simulink model "AutoDriveTest"  (R2023a)
settings: Solver=FixedStepDiscrete  StartTime=0.0  StopTime=10.0  RelTol=1e-3
model workspace (MAT data in the model file):
  firstWarning = 1
  originalScenarioChecksum = '0FA6558D509BC7BD481F436FBA94739B'
libraries: sim3dlib x1, sim3dautolib x1
settings Model: Creator=Franz  LastModifiedBy=Franz

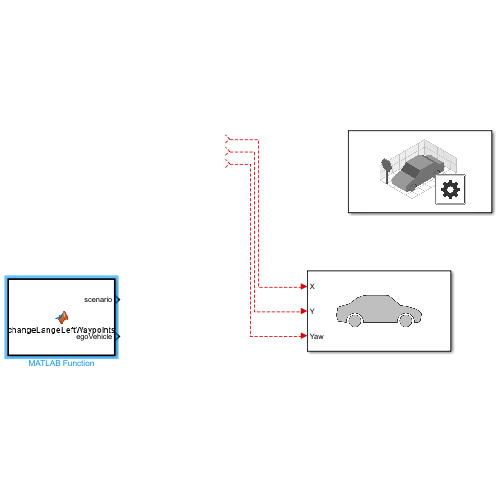
[thumbnail: Simulink's stored preview of the top-level diagram]
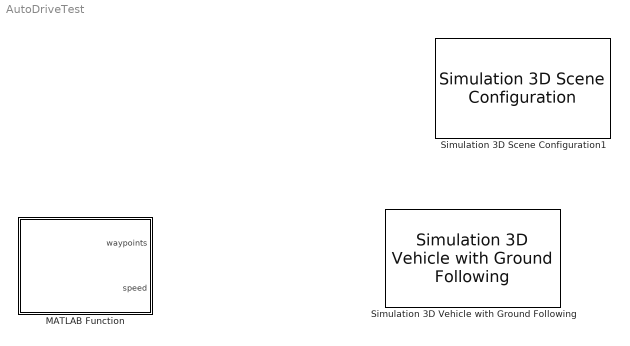
== system AutoDriveTest ==
  MATLAB Function : MATLAB Function  TreatAsAtomicUnit=on
  Simulation 3D Scene Configuration1 : sim3dlib/Simulation 3D Scene Configuration  Priority=0  ProjectFormat=Default Scenes  SceneDesc=Straight road  ProjectName=D:\Program Files\MATLAB\R2023a\toolbox\shared\sim3d_projects\automotive_project\UE4\WindowsNoEditor\VehicleSimulation.exe  ScenePath=/Game/Maps/HwStrght  EnableOpenDRIVE=off  vehTagList={'Scene Origin';'SimulinkVehicle1'}  vehTag=SimulinkVehicle1  OpVisEn=off  Ts=1/60  EnableWindow=off  EnableRemoteAccess=off  EnableWeather=off  SunAltitude=40.0  SunAzimuth=90  clouds=10  wind=1  fog=0  rain=0  EnableGeospatial=off  OriginHeight=200  OriginLatitude=40.744652  OriginLongitude=-73.988864  MapStyle=Aerial  AdditionalAssetIDs=[]  UseAdvancedSunSky=off  SolarTime=11  TimeZone=-5  Day=21  Month=9  Year=2022  UseDaylightSavingTime=on  DSTStartDay=10  DSTStartMonth=3  DSTEndDay=3  DSTEndMonth=11  DSTSwitchHour=2  sensorTag=MainCamera1  sensorId=1  sensorName=MainCamera1  mountLoc=Origin  offsetFlag=off  tmountOffset=[0, 0, 0]  rmountOffset=[0, 0, 0]  HorizontalResolution=1280  VerticalResolution=720  HorizontalFOV=60  mountPoint=[0 0 0]  mountOrientation=[0 0 0]  aMode=3  ID=1  GeoTrigger=Inactive
      settings: LibrarySourceBlock=drivingsim3d/Simulation 3D Scene Configuration
  Simulation 3D Vehicle with Ground Following : sim3dautolib/Simulation 3D Vehicle with Ground Following  Priority=-1  PassVehMesh=Muscle car  MeshPath=/MathWorksAutomotiveContent/Vehicles/Muscle/Meshes/SK_MuscleCar.SK_MuscleCar  TrackWidth=1.9  WheelBase=3  WheelRadius=0.35  VehColor=Red  InitialPos=[0, 0, 0]  InitialRot=[0, 0, 0]  ActorName=SimulinkVehicle1  SampleTime=-1  ActorType=SimulinkVehicle  ID=1  aMode=3  ActorTag=SimulinkVehicle1  CoordinateScheme=ISO  VehLightsControl=off  HeadlightColor=[ 1, 1, 1 ]  HighBeamIntensity=100000  LowBeamIntensity=60000  HighBeamConeAngle=70  LowBeamConeAngle=70  LeftHeadlightOrientation=[ 0, 0 ]  RightHeadlightOrientation=[ 0, 0 ]  BrakelightIntensity=500  ReverselightIntensity=500  SignallightIntensity=500  SignallightPeriod=1  SignalPulseWidth=50  TransformOutportEnabled=off
      settings: LibrarySourceBlock=drivingsim3d/Simulation 3D Vehicle with Ground Following
  wires:
  ? -> Simulation 3D Vehicle with Ground Following/1
  ? -> Simulation 3D Vehicle with Ground Following/2
  ? -> Simulation 3D Vehicle with Ground Following/3

== matlab function AutoDriveTest/MATLAB Function ==
  data: waypoints output; speed output
function [waypoints, speed] = changeLangeLeftWaypoints()
% createDrivingScenario Returns the drivingScenario defined in the Designer

% Generated by MATLAB(R) 9.14 (R2023a) and Automated Driving Toolbox 3.7 (R2023a).
% Generated on: 09-Aug-2023 13:02:59

waypoints = [-5.93127627606 -2.20895520317019 0;
    5.3 -1.6 0;
    14.8 0.9 0;
    24.7 1.4 0;
    33.7 1.4 0];
speed = [50;50;50;50;50];
waittime = [0;0;0;0;0];
trajectory(egoVehicle, waypoints, speed, waittime);
